simulink model "Steeringsystem1"  (R2024a)
settings: Solver=VariableStepAuto  StartTime=0.0  StopTime=5  RelTol=1e-3
libraries: fl_lib x17, nesl_utility x11, ee_lib x1, sdl_lib x1
settings Model: Creator=jesus  LastModifiedBy=kamal

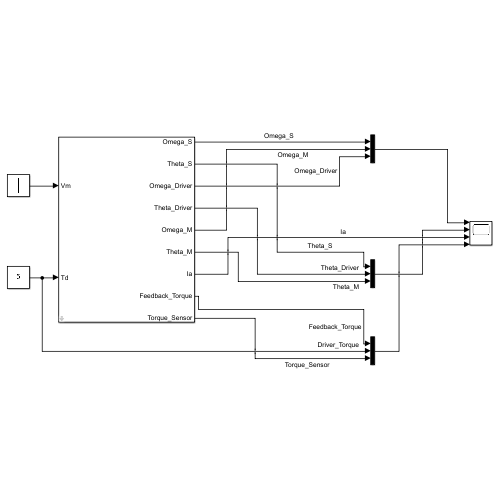
[thumbnail: Simulink's stored preview of the top-level diagram]
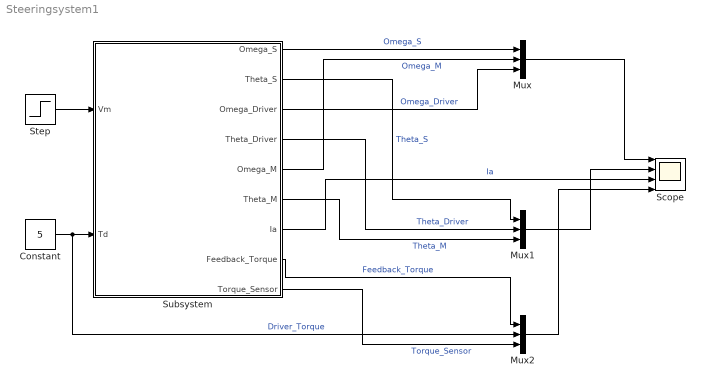
== system Steeringsystem1 ==
  Constant : Constant  Value=5
  Mux : Mux  Inputs=3
  Mux1 : Mux  Inputs=3
  Mux2 : Mux  Inputs=3
  Scope : Scope  NumInputPorts=4
  Step : Step  After=6  SampleTime=0
  Subsystem : Subsystem  mask{Js=0.0012, Bs=0.26, Ks=115, Jm=0.0004704, Bm=0.003339, Im=7.225, Ra=0.1, La=0.1e-3, Ke=0.01}
      mask prompts: Js "Steering column inertia"; Bs "Steering column friction"; Ks "Torsion bar stiffness"; Jm "Motor inertia"; Bm "Motor friction"; Im "Gearbox reduction ratio"; Ra "Armature resistance"; La "Armature inductance"; Ke "Back-emf"
  wires:
  Constant/1 -> Mux2/2, Subsystem/2(Td)  "Driver_Torque"
  Step/1 -> Subsystem/1(Vm)
  Subsystem/1(Omega_S) -> Mux/1  "Omega_S"
  Subsystem/5(Omega_M) -> Mux/2  "Omega_M"
  Subsystem/3(Omega_Driver) -> Mux/3  "Omega_Driver"
  Subsystem/2(Theta_S) -> Mux1/1  "Theta_S"
  Subsystem/4(Theta_Driver) -> Mux1/2  "Theta_Driver"
  Subsystem/6(Theta_M) -> Mux1/3  "Theta_M"
  Mux/1 -> Scope/1
  Mux1/1 -> Scope/2
  Subsystem/7(Ia) -> Scope/3  "Ia"
  Subsystem/8(Feedback_Torque) -> Mux2/1  "Feedback_Torque"
  Mux2/1 -> Scope/4
  Subsystem/9(Torque_Sensor) -> Mux2/3  "Torque_Sensor"

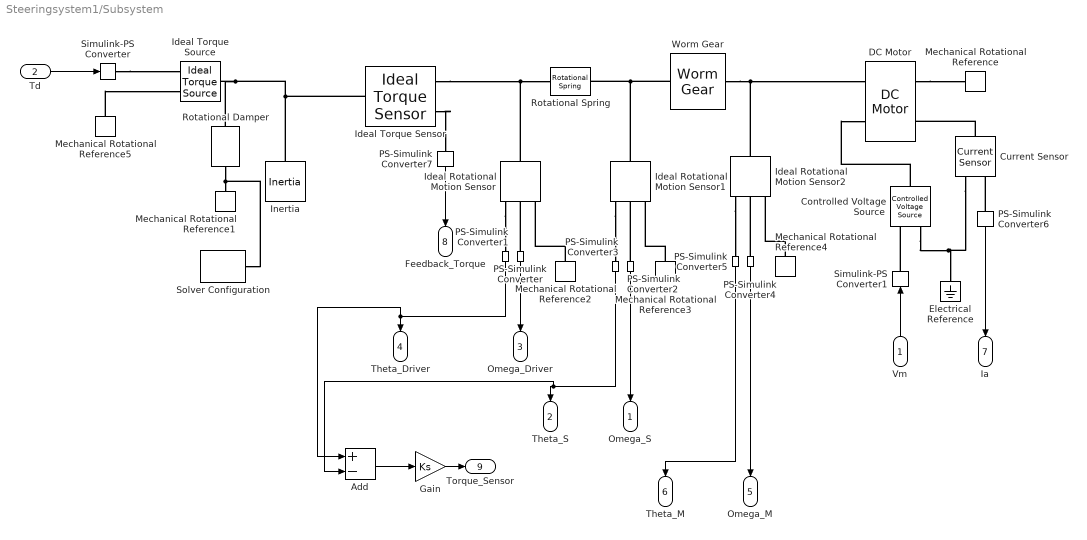
== system Steeringsystem1/Subsystem ==
  Vm : Inport
  Td : Inport  Port=2
  Add : Sum  Inputs=+-
  Controlled Voltage Source : fl_lib/Electrical/Electrical Sources/Controlled Voltage Source
  Current Sensor : fl_lib/Electrical/Electrical Sensors/Current Sensor
  DC Motor : ee_lib/Electromechanical/Brushed Motors/DC Motor  field_option=ee.enum.field_option.pm  Rf=100 Ohm  Lf=1 H  Laf=0.15 H  If0=0 A  parameterization=ee.enum.dcparam_option.circuit_param  Ra=Ra Ohm  La=La H  emf_or_torque=ee.enum.emf_or_torque.kv  Kv=Ke V/rpm  Ki=6.876e-4 N*m/A  T_stall=0.24e-3 N*m  w_max=19100 rpm  w_rated=15000 rpm  P_rated=0.08 W  V_rated=1.5 V  lam_param=ee.enum.lam_param.damping  i_noload=0 A  V_i_noload=1.5 V  J=Jm kg*m^2  lam=Bm N*m*s/rad  speed0=0 rpm  enable_fault_armature=simscape.enum.onoff.off  rev_faulted=1 / 3  G_faulted_armature=1e-5 S  fault_trigger_armature=ee.enum.faults.faultTrigger.temporal  t_fault_armature=1 s  max_permissible_current_armature=inf A  t_fail_on_current_armature=1 s  enable_fault_field=simscape.enum.onoff.off  G_faulted_field=1e-5 S  fault_trigger_field=ee.enum.faults.faultTrigger.temporal  t_fault_field=1 s  max_permissible_current_field=inf A  t_fail_on_current_field=1 s  fault_action=simscape.enum.assert.action.none  alpha=3.93e-3 1/K  Tmeas=25 degC  thermal_mass=100 J/K  initial_temperature=25 degC
  Electrical Reference : fl_lib/Electrical/Electrical Elements/Electrical Reference
  Gain : Gain  Gain=Ks
  Ideal Rotational Motion Sensor : fl_lib/Mechanical/Mechanical Sensors/Ideal Rotational Motion Sensor  reference=foundation.enum.MeasurementReference.difference  acceleration_port=false  velocity_port=true  position_port=true  wrap_angle=false  offset=0 rad
  Ideal Rotational Motion Sensor1 : fl_lib/Mechanical/Mechanical Sensors/Ideal Rotational Motion Sensor  reference=foundation.enum.MeasurementReference.difference  acceleration_port=false  velocity_port=true  position_port=true  wrap_angle=false  offset=0 rad
  Ideal Rotational Motion Sensor2 : fl_lib/Mechanical/Mechanical Sensors/Ideal Rotational Motion Sensor  reference=foundation.enum.MeasurementReference.difference  acceleration_port=false  velocity_port=true  position_port=true  wrap_angle=false  offset=0 rad
  Ideal Torque Sensor : fl_lib/Mechanical/Mechanical Sensors/Ideal Torque Sensor
  Ideal Torque Source : fl_lib/Mechanical/Mechanical Sources/Ideal Torque Source
  Inertia : fl_lib/Mechanical/Rotational Elements/Inertia  inertia=Js kg*m^2  num_ports=foundation.enum.numPorts2.one  w_specify=off  w_priority=High  w=0 rad/s  w_nominal_specify=off  w_nominal_value=1  w_nominal_unit=rad/s  t_specify=off  t_priority=None  t=0 N*m  t_nominal_specify=off  t_nominal_value=1  t_nominal_unit=N*m
  Mechanical Rotational Reference{,1..5} (6 alike) : fl_lib/Mechanical/Rotational Elements/Mechanical Rotational Reference
  PS-Simulink Converter{,1..7} (8 alike) : nesl_utility/PS-Simulink Converter  PhysicalDomain=network_engine_domain  SubClassName=ps_output  LeftPortType=input  RightPortType=output  PseudoPeriodic=off  Frequencies=[]  VectorFormat=inherit  Unit=inherit  AffineConversion=off
  Rotational Damper : fl_lib/Mechanical/Rotational Elements/Rotational Damper  D=Bs N*m*s/rad  w_specify=off  w_priority=None  w=0 rad/s  w_nominal_specify=off  w_nominal_value=1  w_nominal_unit=rad/s  t_specify=off  t_priority=None  t=0 N*m  t_nominal_specify=off  t_nominal_value=1  t_nominal_unit=N*m
  Rotational Spring : fl_lib/Mechanical/Rotational Elements/Rotational Spring  spr_rate=Ks N*m/rad  w_specify=off  w_priority=None  w=0 rad/s  w_nominal_specify=off  w_nominal_value=1  w_nominal_unit=rad/s  t_specify=off  t_priority=None  t=0 N*m  t_nominal_specify=off  t_nominal_value=1  t_nominal_unit=N*m  phi_specify=off  phi_priority=High  phi=0 rad  phi_nominal_specify=off  phi_nominal_value=1  phi_nominal_unit=rad
  Simulink-PS Converter : nesl_utility/Simulink-PS Converter  PhysicalDomain=network_engine_domain  SubClassName=ps_input  LeftPortType=input  RightPortType=output  PseudoPeriodic=off  Frequencies=[]  NoiseDistribution=none  NoiseParameters=[]  Unit=1  AffineConversion=off  FilteringAndDerivatives=provide  SimscapeFilterOrder=1  InputFilterTimeConstant=0.001  UdotUserProvided=0
  Simulink-PS Converter1 : nesl_utility/Simulink-PS Converter  PhysicalDomain=network_engine_domain  SubClassName=ps_input  LeftPortType=input  RightPortType=output  PseudoPeriodic=off  Frequencies=[]  NoiseDistribution=none  NoiseParameters=[]  Unit=1  AffineConversion=off  FilteringAndDerivatives=provide  SimscapeFilterOrder=1  InputFilterTimeConstant=0.001  UdotUserProvided=0
  Solver Configuration : nesl_utility/Solver Configuration  PhysicalDomain=network_engine_domain  SubClassName=solver  LeftPortType=input  RightPortType=generic  Tones=[]  Harmonics=[]  SimulateNoise=off  Profile=off  UseLocalSampling=off  EnableSwitchedLinearOptims=on  FrequencyDomain=off  UseCCode=off  RelTol=0.001  AbsTol=0.001  MinStep=1e-09  ToWorkspace=off  RevertToSquareIcSolve=off  NumHomotopyIterations=100  PhasorMode=off  PhasorModeNumHarmonics=1  ConsistencySolver=NEWTON_XTOL_AFTER_FTOL  IndexReductionMethod=DerivativeReplacement  DoDC=off  ResidualTolerance=1e-09  ConsistencyTolSource=GLOBAL  ConsistencyAbsTol=0.001  ConsistencyRelTol=0.001  ConsistencyTolFactor=0.001  UseLocalSolver=off  LocalSolverChoice=NE_BACKWARD_EULER_ADVANCER  ResolveIndetEquations=on  FunctionEvalNumThread=1  LocalSolverSampleTime=0.001  DoFixedCost=off  MaxNonlinIter=3  MaxModeIter=2  ComputeImpulses=off  ImpulseIterations=2  LinearAlgebra=auto  LinearAlgebraNumThread=0  EquationFormulation=NE_TIME_EF  DelaysMemoryBudget=1024  AutomaticFiltering=on  FilteringTimeConstant=0.001  PartitionStorageMethod=AS_NEEDED  PartitionMemoryBudget=1024  PartitionMethod=ROBUST  MultibodyUseLocalSolver=off  MultibodyLocalSolverChoice=ODE1  MultibodyLocalSolverSampleTime=0.001
  Worm Gear : sdl_lib/Gears/Worm Gear  ratio=Im  thread_type=sdl.enum.handedness.left  friction_model=sdl.enum.gear_friction.none  friction_parameterization=sdl.enum.efficiency_geometry.geometry  pr_ang=17.5 deg  lead_ang=20 deg  fr_coeff=0.08  eff_wg=0.74  eff_gw=0.65  temperature_TLU=[280, 300, 320] K  efficiency_wg_TLU=[.75, .65, .6]  efficiency_gw_TLU=[.5, .45, .4]  pwr_thr=0.001 W  mu_visc=[0, 0] N*m*s/rad  thermal_mass=50 J/K  temperature_specify=off  temperature_priority=High  temperature=300 K  temperature_nominal_specify=off  temperature_nominal_value=1  temperature_nominal_unit=K
      settings: InternalSimscapePortConfiguration="{\"Bottom\":[],\"Left\":[{\"id\":\"W\",\"label\":\"W\",\"type\":\"foundation.mechanical.rotational.rotational\"}],\"Right\":[{\"id\":\"G\",\"label\":\"G\",\"type\":\"foundation.mechanical.rotational.rotational\"}],\"Top\":[]}"
  Omega_S : Outport
  Theta_S : Outport  Port=2
  Omega_Driver : Outport  Port=3
  Theta_Driver : Outport  Port=4
  Omega_M : Outport  Port=5
  Theta_M : Outport  Port=6
  Ia : Outport  Port=7
  Feedback_Torque : Outport  Port=8
  Torque_Sensor : Outport  Port=9
  wires:
  PS-Simulink Converter2/1 -> Omega_S/1
  PS-Simulink Converter1/1 -> Add/1, Theta_Driver/1
  Td/1 -> Simulink-PS Converter/1
  PS-Simulink Converter/1 -> Omega_Driver/1
  PS-Simulink Converter3/1 -> Add/2, Theta_S/1
  PS-Simulink Converter4/1 -> Omega_M/1
  PS-Simulink Converter6/1 -> Ia/1
  PS-Simulink Converter5/1 -> Theta_M/1
  Vm/1 -> Simulink-PS Converter1/1
  PS-Simulink Converter7/1 -> Feedback_Torque/1
  Add/1 -> Gain/1
  Gain/1 -> Torque_Sensor/1
  connections:
  Controlled Voltage Source/RConn2 -- Current Sensor/RConn2 -- Electrical Reference/LConn1
  PS-Simulink Converter2/LConn1 -- Ideal Rotational Motion Sensor1/RConn2
  Inertia/LConn1 -- Ideal Torque Sensor/LConn1 -- Rotational Damper/LConn1 -- Ideal Torque Source/LConn1
  Worm Gear/LConn1 -- Ideal Rotational Motion Sensor2/LConn1 -- DC Motor/LConn2
  Simulink-PS Converter1/RConn1 -- Controlled Voltage Source/RConn1
  Current Sensor/LConn1 -- DC Motor/RConn1
  Mechanical Rotational Reference3/LConn1 -- Ideal Rotational Motion Sensor1/RConn1
  Ideal Rotational Motion Sensor/LConn1 -- Ideal Torque Sensor/RConn1 -- Rotational Spring/LConn1
  PS-Simulink Converter4/LConn1 -- Ideal Rotational Motion Sensor2/RConn2
  PS-Simulink Converter/LConn1 -- Ideal Rotational Motion Sensor/RConn2
  Ideal Rotational Motion Sensor2/RConn3 -- PS-Simulink Converter5/LConn1
  Worm Gear/RConn1 -- Ideal Rotational Motion Sensor1/LConn1 -- Rotational Spring/RConn1
  Rotational Damper/RConn1 -- Solver Configuration/RConn1 -- Mechanical Rotational Reference1/LConn1
  Mechanical Rotational Reference2/LConn1 -- Ideal Rotational Motion Sensor/RConn1
  Mechanical Rotational Reference4/LConn1 -- Ideal Rotational Motion Sensor2/RConn1
  DC Motor/RConn2 -- Mechanical Rotational Reference/LConn1
  Simulink-PS Converter/RConn1 -- Ideal Torque Source/RConn1
  Ideal Rotational Motion Sensor/RConn3 -- PS-Simulink Converter1/LConn1
  Ideal Rotational Motion Sensor1/RConn3 -- PS-Simulink Converter3/LConn1
  Ideal Torque Sensor/RConn2 -- PS-Simulink Converter7/LConn1
  Controlled Voltage Source/LConn1 -- DC Motor/LConn1
  PS-Simulink Converter6/LConn1 -- Current Sensor/RConn1
  Mechanical Rotational Reference5/LConn1 -- Ideal Torque Source/RConn2
